simulink model "auto_pilot_udp"  (R2022b)
settings: Solver=FixedStepAuto  StartTime=0.0  StopTime=Inf  FixedStep=0.001  RelTol=1e-3  EnableMultiTasking=on
InitFcn:
  | clear mex
model workspace (MAT data in the model file):
  worldsim_instance.endpoint_ip = '127.0.0.1'
  worldsim_instance.endpoint_port = 8080
values from neighbouring files (symbols this model uses):
  ACC_Adaptive_D = 0    [AutoPilot_parameters.m]    (also in ap_ini_param.mat; ap_initialModel.sldd = 0.0)
  ACC_Adaptive_I = 0    [AutoPilot_parameters.m]    (also in ap_ini_param.mat; ap_initialModel.sldd = 0.0)
  ACC_Adaptive_P = [5 7.5]    [AutoPilot_parameters.m]    (also in ap_ini_param.mat; ap_initialModel.sldd = 5.0 7.5)
  ACC_Classic_I = 5    [AutoPilot_parameters.m]    (also in ap_ini_param.mat; ap_initialModel.sldd = 5.0)
  ACC_Classic_P = 15    [AutoPilot_parameters.m]    (also in ap_ini_param.mat; ap_initialModel.sldd = 15.0)
  ACC_MaxBrake = 50    [AutoPilot_parameters.m]    (also in ap_ini_param.mat; ap_initialModel.sldd = 50.0)
  ACC_MaxThrottle = 130    [AutoPilot_parameters.m]    (also in ap_ini_param.mat = 80; ap_initialModel.sldd = 130.0)
  ACC_Module_Activity_Flag = 1    [AutoPilot_parameters.m]    (also in ap_ini_param.mat; ap_initialModel.sldd = 1.0)
  ACC_Ready_Speed = 30    [AutoPilot_parameters.m]    (also in ap_ini_param.mat; ap_initialModel.sldd = 30.0)
  ACC_SensorMaxDistance = 250    [AutoPilot_parameters.m]    (also in ap_ini_param.mat = 120; ap_initialModel.sldd = 250.0)
  ACC_Speed_Distance_control = 3    [AutoPilot_parameters.m]    (also in ap_ini_param.mat; ap_initialModel.sldd = 3.0)
  ACC_Speed_Distance_Gain = [0.1 0.15 0.2 0.25]    [AutoPilot_parameters.m]    (also in ap_ini_param.mat; ap_initialModel.sldd = 0.1 0.15 0.2 0.25)
  ADAS_Control_Mode = 1    [AutoPilot_parameters.m]    (also in ap_ini_param.mat; ap_initialModel.sldd = 1.0)
  AEB_Alarm_Freq = 5    [AutoPilot_parameters.m]    (also in ap_ini_param.mat; ap_initialModel.sldd = 5.0)
  AEB_Distance_To_Collision_Brake = 5    [AutoPilot_parameters.m]    (also in ap_ini_param.mat; ap_initialModel.sldd = 5.0)
  AEB_Freq_Hz = Sensor_Freq_worldsim/2    (= 25)    [AutoPilot_parameters.m]    (also in ap_ini_param.mat; ap_initialModel.sldd = 25.0)
  AEB_Gain = [1 1]    [AutoPilot_parameters.m]    (also in ap_ini_param.mat; ap_initialModel.sldd = 1.0 1.0)
  AEB_Gain_set = 60    [AutoPilot_parameters.m]    (also in ap_ini_param.mat; ap_initialModel.sldd = 60.0)
  AEB_Gain_set_mult = 0.03    [AutoPilot_parameters.m]    (also in ap_ini_param.mat; ap_initialModel.sldd)
  AEB_Max_Decel = [8 15]    [AutoPilot_parameters.m]    (also in ap_ini_param.mat; ap_initialModel.sldd = 8.0 15.0)
  AEB_Max_Speed = 150    [AutoPilot_parameters.m]    (also in ap_ini_param.mat = 100; ap_initialModel.sldd = 150.0)
  AEB_Min_Distance_at_Stop = 1    [AutoPilot_parameters.m]    (also in ap_ini_param.mat; ap_initialModel.sldd = 1.0)
  AEB_Module_Activity_Flag = 1    [AutoPilot_parameters.m]    (also in ap_ini_param.mat; ap_initialModel.sldd = 1.0)
  AEB_Pedestrian_type = 68    [AutoPilot_parameters.m]    (also in ap_ini_param.mat; ap_initialModel.sldd = 68.0)
  AEB_Steer_Max = 180    [AutoPilot_parameters.m]    (also in ap_ini_param.mat; ap_initialModel.sldd = 180.0)
  AP_Activity_Flag = 1    [AutoPilot_parameters.m]    (also in ap_ini_param.mat; ap_initialModel.sldd = 1.0)
  AP_D = [0.3 0.3]    [AutoPilot_parameters.m]    (also in ap_ini_param.mat; ap_initialModel.sldd = 0.3 0.3)
  AP_Dyn_Rate_Limiter_Gain = 0.1    [AutoPilot_parameters.m]    (also in ap_ini_param.mat; ap_initialModel.sldd)
  AP_Dyn_Rate_Limiter_Power = 10    [AutoPilot_parameters.m]    (also in ap_ini_param.mat; ap_initialModel.sldd = 10.0)
  AP_Error_Max = 3    [AutoPilot_parameters.m]    (also in ap_ini_param.mat; ap_initialModel.sldd = 3.0)
  AP_Freq_Hz = Sensor_Freq_worldsim    (= 50)    [AutoPilot_parameters.m]    (also in ap_ini_param.mat; ap_initialModel.sldd = 50.0)
  AP_I = [0.05 0.05]    [AutoPilot_parameters.m]    (also in ap_ini_param.mat; ap_initialModel.sldd = 0.05 0.05)
  AP_Max_Error_dydt_Disable = 0.5    [AutoPilot_parameters.m]    (also in ap_ini_param.mat; ap_initialModel.sldd)
  AP_On_Request_Time = 0.01    [AutoPilot_parameters.m]    (also in ap_ini_param.mat; ap_initialModel.sldd)
  AP_P = [0.2 0.2]    [AutoPilot_parameters.m]    (also in ap_ini_param.mat; ap_initialModel.sldd = 0.2 0.2)
  AP_Steer_Error_Max = 0.7    [AutoPilot_parameters.m]    (also in ap_ini_param.mat; ap_initialModel.sldd)
  AP_Steer_Rate_Max_radps = 1    [AutoPilot_parameters.m]    (also in ap_ini_param.mat; ap_initialModel.sldd = 1.0)
  AP_Transition_Rate = 0.5    [AutoPilot_parameters.m]    (also in ap_ini_param.mat; ap_initialModel.sldd)
  butter_a = [1 -1.9911142922 0.991153595869]    [ap_ini_param.mat]    (also in ap_initialModel.sldd = 1.0 -1.9911142922016536 0.99115359586893548)
  butter_a_lka_out = 1.0 -1.5610180758007179 0.641351538057563    [ap_initialModel.sldd]
  butter_b = [9.82591682048e-06 1.9651833641e-05 9.82591682048e-06]    [ap_ini_param.mat]    (also in ap_initialModel.sldd = 9.825916820482009E-6 1.9651833640964018E-5 9.825916820482009)
  butter_b_lka_out = 0.020083365564211246 0.040166731128422492 0.020083365564211246    [ap_initialModel.sldd]
  Lane_Width = 3.7    [AutoPilot_parameters.m]    (also in ap_ini_param.mat; ap_initialModel.sldd)
  LDW_Activity_Flag = 1    [ap_ini_param.mat]    (also in ap_initialModel.sldd = 1.0)
  LDW_Freq_Hz = 50    [ap_ini_param.mat]    (also in ap_initialModel.sldd = 50.0)
  LDW_LaneGap_dydt_Warning = 50    [ap_ini_param.mat]    (also in ap_initialModel.sldd = 50.0)
  LDW_LaneGap_Warning = [0.5 0.25]    [ap_ini_param.mat]    (also in ap_initialModel.sldd = 0.5 0.25)
  LDW_Min_Speed = 60    [ap_ini_param.mat]    (also in ap_initialModel.sldd = 60.0)
  LDW_Steer_Vibration_Amplitude = 5    [ap_ini_param.mat]    (also in ap_initialModel.sldd = 5.0)
  LDW_Steer_Vibration_Freq = 25    [ap_ini_param.mat]    (also in ap_initialModel.sldd = 25.0)
  LKA_Activity_Flag = 1    [ap_ini_param.mat]    (also in ap_initialModel.sldd = 1.0)
  LKA_D = [0.2 0.3]    [ap_ini_param.mat]    (also in ap_initialModel.sldd = 0.2 0.3)
  LKA_Dyn_Rate_Limiter_Gain = 0.1    [ap_ini_param.mat]    (also in ap_initialModel.sldd)
  LKA_Dyn_Rate_Limiter_Power = 10    [ap_ini_param.mat]    (also in ap_initialModel.sldd = 10.0)
  LKA_Error_dydt_Off = 1    [ap_ini_param.mat]    (also in ap_initialModel.sldd = 1.0)
  LKA_Error_Max = 3    [ap_ini_param.mat]    (also in ap_initialModel.sldd = 3.0)
  LKA_Error_Off = 0.5    [ap_ini_param.mat]    (also in ap_initialModel.sldd)
  LKA_Freq_Hz = 50    [ap_ini_param.mat]    (also in ap_initialModel.sldd = 50.0)
  LKA_I = [0.025 0.05]    [ap_ini_param.mat]    (also in ap_initialModel.sldd = 0.025 0.05)
  LKA_Lane_Gap_Activate = [0.25 0.125]    [ap_ini_param.mat]    (also in ap_initialModel.sldd = 0.25 0.125)
  LKA_Lane_Gap_dydt_Activate = 50    [ap_ini_param.mat]    (also in ap_initialModel.sldd = 50.0)
  LKA_Min_Speed = 60    [ap_ini_param.mat]    (also in ap_initialModel.sldd = 60.0)
  LKA_On_Display_Freq = 5    [ap_ini_param.mat]    (also in ap_initialModel.sldd = 5.0)
  LKA_P = [0.1 0.2]    [ap_ini_param.mat]    (also in ap_initialModel.sldd = 0.1 0.2)
  LKA_Steer_Rate_Max_radps = 1    [ap_ini_param.mat]    (also in ap_initialModel.sldd = 1.0)
  No_Target_Display_Value = 0    [AutoPilot_parameters.m]    (also in ap_ini_param.mat; ap_initialModel.sldd = 0.0)
  radar_source = 2    [AutoPilot_parameters.m]    (also in ap_ini_param.mat; ap_initialModel.sldd = 2.0)
  Sensor_Freq_worldsim = 50    [AutoPilot_parameters.m]    (also in ap_ini_param.mat; ap_initialModel.sldd = 50.0; launcher.m)
  stop_number_collisions = 10.0    [ap_initialModel.sldd]    (also in launcher.m = 10)
  stop_speed = 0.001    [ap_initialModel.sldd]    (also in launcher.m)
  stop_time = 12.0    [ap_initialModel.sldd]    (also in launcher.m = 12)
  vehicle_width = 2.2    [AutoPilot_parameters.m]    (also in ap_ini_param.mat = 1.86; ap_initialModel.sldd)
undefined symbols (not defined in the file or in its folder): blockPlatform, HOST, light_brake_center, light_brake_left, light_brake_right
libraries: simulink x103, simwbSfunlib x35, slpidlib x5, viworldsim_lib x5
(part 1 of 5)
settings Model: DataDictionary=ap_initialModel.sldd  Creator=mcava  LastModifiedBy=pumpaipa
settings SolverCC: AlgebraicLoopSolver=TrustRegion  AutoInsertRateTranBlk=on
settings DataIOCC: LimitDataPoints=on  SaveFormat=Array  ReturnWorkspaceOutputs=off  SignalLoggingName=sigsOut
settings OptimizationCC: ExpressionDepthLimit=2147483647  InitFltsAndDblsToZero=on
settings DebuggingCC: SignalInfNanChecking=warning  UnderspecifiedInitializationDetection=Classic  MergeDetectMultiDrivingBlocksExec=none  SignalResolutionControl=TryResolveAllWithWarning  MultiTaskDSMMsg=warning  MultiTaskCondExecSysMsg=none  FcnCallInpInsideContextMsg=warning  UnconnectedInputMsg=warning  UnconnectedOutputMsg=warning  UnconnectedLineMsg=warning  StateNameClashWarn=warning  SFUnexpectedBacktrackingDiag=warning  SFNoUnconditionalDefaultTransitionDiag=warning  SFExecutionAtInitializationDiag=none  SFMachineParentedDataDiag=warning  ArithmeticOperatorsInVariantConditions=warning
settings HardwareCC: ProdBitPerLong=64  ProdHWDeviceType=Intel->x86-64 (Linux 64)  TargetHWDeviceType=32-bit Generic
settings ModelReferenceCC: EnableRefExpFcnMdlSchedulingChecks=on  PropagateSignalLabelsOutOfModel=off
settings SFSimCC: SimUseLocalCustomCode=off  CustomCodeUndefinedFunction=UseInterfaceOnly
settings RTWCC: Description=VI-CarRealTime Solver Plugin V1.0  SystemTargetFile=vicrt_plugin.tlc  GenCodeOnly=on  PackageGeneratedCodeAndArtifacts=on  TemplateMakefile=vicrt_plugin_ccur.tmf  PostCodeGenCommand=if strcmp(get_param(bdroot,'TemplateMakefile'),'vicrt_plugin_ccur.tmf'),copyfile([matlabroot,filesep,'rtw',filesep,'c',filesep,'tools',filesep,'unixtools.mk'],'unixtools.mk'),if ~verLessThan('matlab','9.6'),set_param(bdroot,'MatFileLogging','off'),end,end  RTWUseLocalCustomCode=off
settings CodeAppCC: MaxIdLength=80  StateflowObjectComments=on
settings STFCustomTargetCC: ModelReferenceCompliant=off  CombineOutputUpdateFcns=on  SystemTargetFile=vicrt_plugin.tlc
settings GRTTargetCC: TargetLangStandard=C89/C90 (ANSI)  ModelReferenceCompliant=off  ParMdlRefBuildCompliant=off  CompOptLevelCompliant=off  ConcurrentExecutionCompliant=off  MatFileLogging=off  CPPClassGenCompliant=off  UseToolchainInfoCompliant=off  RTWCAPIParams=on
settings ConfigComp: CovMetricSettings=dw  CovSaveCumulativeToWorkspaceVar=on  CovSaveSingleToWorkspaceVar=on  CovExternalEMLEnable=off

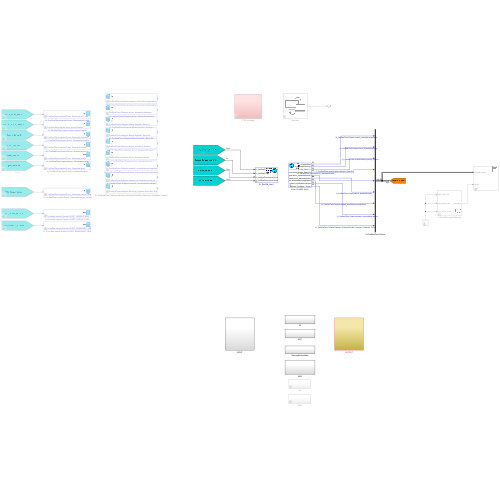
[thumbnail: Simulink's stored preview of the top-level diagram]
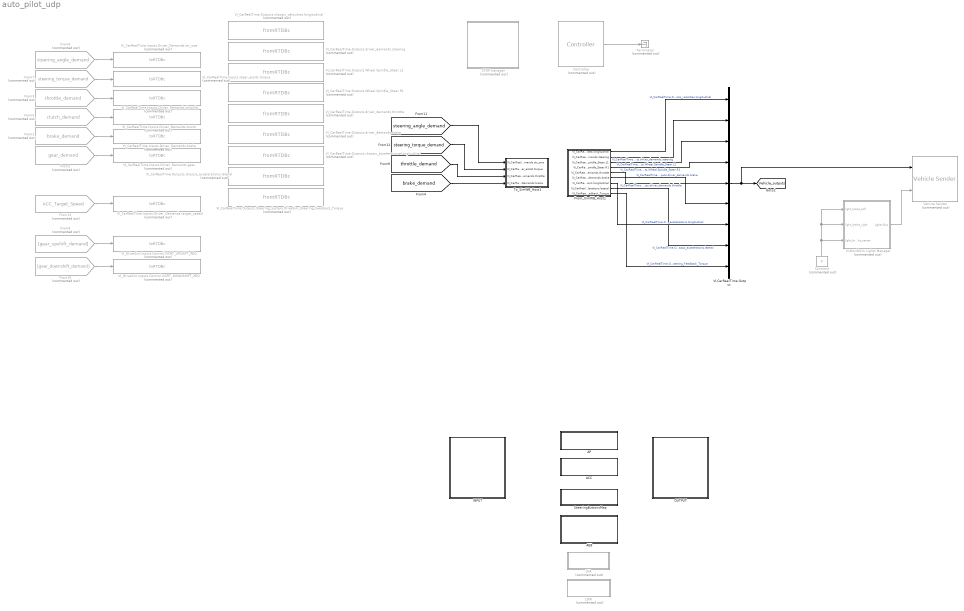
== system auto_pilot_udp ==
  ACC : Subsystem
  AEB : Subsystem
  AP : Subsystem
  Constant : Constant  Commented=on  Value=0
  Controller : viworldsim_lib/Controller  Commented=on  worldsim_endpoint_ip=worldsim_instance.endpoint_ip  worldsim_endpoint_port=worldsim_instance.endpoint_port  worldsim_verbose=off
  From1 : From  Commented=on  GotoTag=brake_demand  TagVisibility=global
  From10 : From  Commented=on  GotoTag=gear_downshift_demand  TagVisibility=global
  From13 : From  Commented=on  GotoTag=ACC_Target_Speed  TagVisibility=global
  From2 : From  Commented=on  GotoTag=gear_demand  TagVisibility=global
  From3 : From  Commented=on  GotoTag=throttle_demand  TagVisibility=global
  From5 : From  Commented=on  GotoTag=clutch_demand  TagVisibility=global
  From6 : From  Commented=on  GotoTag=steering_angle_demand  TagVisibility=global
  From7 : From  Commented=on  GotoTag=steering_torque_demand  TagVisibility=global
  From8 : From  Commented=on  GotoTag=gear_upshift_demand  TagVisibility=global
  From_SimWB_Host1 : Subsystem  mask(From_SimWB_Host){numPorts=9, inheritPortNames=off, portNames={'VI_CarRealTime.Outputs.chassis_velocities.longitudinal','VI_CarRealTime.Outputs.driver_demands.steering','VI_CarRealTime.Outputs.Wheel.Spindle_Steer.L1','VI_CarRealTime.Outputs.Wheel.Spindle_Steer.R1','VI_CarRealTime.Outputs.driver_demands.throttle','VI_CarRealTime.Outputs.driver_demands.brake','VI_CarRealTime.Outputs.chassis_accelerations.longitudinal','VI_CarRealTime.Outputs.chassis_accelerations.lateral','VI_CarRealTime.Outputs.Steering_System.DriveSim_Steering_Feedback_Torque'}, origNumPorts=1, blockCode=6578738372in, localIP='192.168.100.150', localPort=25000, remoteURL='192.168.100.20', recvBufferSize=72, dims=72, blockingTime=0, sampletime=0.01, signalDatatype=uint8, isVarSize=off, blockPlatform=blockPlatform, isComplex=on, msk_dimensions={1,1,1,1,1,1,1,1,1}, msk_datatypes={'double','double','double','double','double','double','double','double','double'}, byteAlign=1}
      mask prompts: numPorts "Number of Ports:"; inheritPortNames "Inherit Port Names:"; portNames "Port Names: {'a','b','c'}"; origNumPorts "Orig Num"; blockCode "Block Code"; localIP "Local IP address (SimWB sends data to this IP)"; localPort "Local IP port:"; remoteURL "Remote IP address ('0.0.0.0' to accept all):"; recvBufferSize "Receive buffer size (bytes):"; dims "Maximum length for Message:"; blockingTime "Blocking time (seconds):"; sampletime "Sample time (seconds):"; signalDatatype "Data type for Message:"; isVarSize "Output variable-size signal"; blockPlatform "Block Platform:"; isComplex "Message is Complex"; msk_dimensions "Output port dimensions:"; msk_datatypes "Output port data type:"; byteAlign "Byte alignment:"
      mask help: This block receives UDP packets from the specified SimWB host. This block is supported in MATLAB R2011a and later only.
      mask init:
      | set_param(gcbh,'blockCode','6578738372in');
      mask Help: web([simwbroot 'html' filesep 'simwb_blocks_udp.html'])
      mask Callback numPorts: UDPBlockSetup(gcbh,'INPUT');
      mask Callback inheritPortNames:
      | maskVisibilities =  get_param(gcbh,'MaskVisibilities');
      | if  strcmp(get_param(gcbh,'inheritPortNames'),'on')
      |     maskVisibilities{3} = 'off';
      | else
      |     maskVisibilities{3} = 'on';
      | end
      | set_param(gcbh,'MaskVisibilities',maskVisibilities);
      mask Callback portNames: UDPBlockSetup(gcbh,'UPDATEOUTPORTNAMES');
      mask Callback msk_dimensions: UDPBlockSetup(gcbh,'BYTEUNPACKCHANGED');
      mask Callback msk_datatypes: UDPBlockSetup(gcbh,'BYTEUNPACKCHANGED');
      mask DialogControl ParameterTabVar0 Prompt: General
      mask DialogControl ParameterTabVar01 Prompt: UDP
      mask DialogControl ParameterTabVar012 Prompt: Byte Unpack
      mask Display: image(imread('udpreceive.png'),'top-left')
  INPUT : Subsystem
  LDW : Subsystem  Commented=on
  LKA : Subsystem  Commented=on
  OUTPUT : Subsystem
  STOP manager : Subsystem  Commented=on
  SteeringButtonsMap : Subsystem
  Terminator : Terminator  Commented=on
  To_SimWB_Host1 : Subsystem  mask(To_SimWB_Host){numPorts=4, inheritPortNames=off, portNames={'VI_CarRealTime.Inputs.Driver_Demands.str_swa','VI_CarRealTime.Inputs.steer_assist.torque','VI_CarRealTime.Inputs.Driver_Demands.throttle','VI_CarRealTime.Inputs.Driver_Demands.brake'}, remoteURL='255.255.255.255', remotePort=25001, blockPlatform=HOST, msk_datatypes={'double','double','double','double'}, byteAlign=1, origNumPorts=1, blockCode=6578738372out, sendBufferSize=8192}
      mask prompts: numPorts "Number of Ports:"; inheritPortNames "Inherit Port Names:"; portNames "Port Names: {'a','b','c'}"; remoteURL "Remote IP address ('255.255.255.255' for broadcast):"; remotePort "Remote IP port:"; blockPlatform "Block Platform"; msk_datatypes "Input port data types (cell array):"; byteAlign "Byte alignment:"; origNumPorts "Orig Num"; blockCode "Block Code"; sendBufferSize "Send Buffer Size"
      mask help: This block sends UDP packets to the specified SimWB host. This block is supported in MATLAB R2011a and later only.
      mask Help: web([simwbroot 'html' filesep 'simwb_blocks_udp.html']);
      mask Callback numPorts: UDPBlockSetup(gcbh,'OUTPUT');
      mask Callback inheritPortNames:
      | maskVisibilities =  get_param(gcbh,'MaskVisibilities');
      | if  strcmp(get_param(gcbh,'inheritPortNames'),'on')
      |     maskVisibilities{3} = 'off';
      | else
      |     maskVisibilities{3} = 'on';
      | end
      | set_param(gcbh,'MaskVisibilities',maskVisibilities);
      mask Callback portNames: UDPBlockSetup(gcbh,'UPDATEINPORTNAMES');
      mask Callback msk_datatypes: UDPBlockSetup(gcbh,'BYTEPACKCHANGED');
      mask DialogControl ParameterTabVar0 Prompt: General
      mask DialogControl ParameterTabVar01 Prompt: UDP
      mask DialogControl ParameterTabVar012 Prompt: Byte Pack
      mask Display: image(imread('udpsend.png'),'top-right')
  VI-CarRealTime.Output : BusCreator  Inputs=9
  VI-WorldSim Lights Manager : Subsystem  Commented=on  mask{DummyMaskPar=0}
      mask init:
      | set_param(gcb, 'LinkStatus','none')
      settings: OpenFcn=|
      | wsoffline_lightsmanager;
      | set_param(gcb, 'LinkStatus','none');
      mask Display:
      | color('black');
      | image('lights.png', [85 0 50 50]);
  VI_CarRealTime.Inputs.Driver_Demands.brake : simwbSfunlib/toRTDBc  Commented=on  stringBlock=off  varName=VI_CarRealTime.Inputs.Driver_Demands.brake  sigDim=[1 1]  sigType=double  sampleTime=[-1 0]  maxBuffSize=1024  busName=nobus  defaultValue=0  defaultString=simwbout  hasMapping=0  ptrName=VI_CarRealTime_Inputs_Driver_Demands_brake  enumOrAlias=nothing
      settings: SourceProductName=SimWB MLToolkit
  VI_CarRealTime.Inputs.Driver_Demands.clutch : simwbSfunlib/toRTDBc  Commented=on  stringBlock=off  varName=VI_CarRealTime.Inputs.Driver_Demands.clutch  sigDim=[1 1]  sigType=double  sampleTime=[-1 0]  maxBuffSize=1024  busName=nobus  defaultValue=0  defaultString=simwbout  hasMapping=0  ptrName=VI_CarRealTime_Inputs_Driver_Demands_clutch  enumOrAlias=nothing
      settings: SourceProductName=SimWB MLToolkit
  VI_CarRealTime.Inputs.Driver_Demands.gear : simwbSfunlib/toRTDBc  Commented=on  stringBlock=off  varName=VI_CarRealTime.Inputs.Driver_Demands.gear  sigDim=[1 1]  sigType=double  sampleTime=[-1 0]  maxBuffSize=1024  busName=nobus  defaultValue=0  defaultString=simwbout  hasMapping=0  ptrName=VI_CarRealTime_Inputs_Driver_Demands_gear  enumOrAlias=nothing
      settings: SourceProductName=SimWB MLToolkit
  VI_CarRealTime.Inputs.Driver_Demands.str_swa : simwbSfunlib/toRTDBc  Commented=on  stringBlock=off  varName=VI_CarRealTime.Inputs.Driver_Demands.str_swa  sigDim=[1 1]  sigType=double  sampleTime=[-1 0]  maxBuffSize=1024  busName=nobus  defaultValue=0  defaultString=simwbout  hasMapping=0  ptrName=VI_CarRealTime_Inputs_Driver_Demands_str_swa  enumOrAlias=nothing
      settings: SourceProductName=SimWB MLToolkit
  VI_CarRealTime.Inputs.Driver_Demands.target_speed : simwbSfunlib/toRTDBc  Commented=on  stringBlock=off  varName=VI_CarRealTime.Inputs.Driver_Demands.target_speed  sigDim=[1 1]  sigType=double  sampleTime=[-1 0]  maxBuffSize=1024  busName=nobus  defaultValue=0  defaultString=simwbout  hasMapping=0  ptrName=VI_CarRealTime_Inputs_Driver_Demands_target_speed  enumOrAlias=nothing
      settings: SourceProductName=SimWB MLToolkit
  VI_CarRealTime.Inputs.Driver_Demands.throttle : simwbSfunlib/toRTDBc  Commented=on  stringBlock=off  varName=VI_CarRealTime.Inputs.Driver_Demands.throttle  sigDim=[1 1]  sigType=double  sampleTime=[-1 0]  maxBuffSize=1024  busName=nobus  defaultValue=0  defaultString=simwbout  hasMapping=0  ptrName=VI_CarRealTime_Inputs_Driver_Demands_throttle  enumOrAlias=nothing
      settings: SourceProductName=SimWB MLToolkit
  VI_CarRealTime.Inputs.steer_assist.torque : simwbSfunlib/toRTDBc  Commented=on  stringBlock=off  varName=VI_CarRealTime.Inputs.steer_assist.torque  sigDim=[1 1]  sigType=double  sampleTime=[-1 0]  maxBuffSize=1024  busName=nobus  defaultValue=0  defaultString=simwbout  hasMapping=0  ptrName=VI_CarRealTime_Inputs_steer_assist_torque  enumOrAlias=nothing
      settings: SourceProductName=SimWB MLToolkit
  VI_CarRealTime.Outputs.Steering_System.DriveSim_Steering_Feedback_Torque : simwbSfunlib/fromRTDBc  Commented=on  stringBlock=off  varName=VI_CarRealTime.Outputs.Steering_System.DriveSim_Steering_Feedback_Torque  sigDim=[1 1]  sigType=double  sampleTime=[-1 0]  maxBuffSize=1024  busName=nobus  defaultValue=0  defaultString=simwbin  hasMapping=0  ptrName=VI_CarRealTime_Outputs_Steering_System_DriveSim_Steering_Feedback_Torque  enumOrAlias=nothing
      settings: SourceProductName=SimWB MLToolkit
  VI_CarRealTime.Outputs.Wheel.Spindle_Steer.L1 : simwbSfunlib/fromRTDBc  Commented=on  stringBlock=off  varName=VI_CarRealTime.Outputs.Wheel.Spindle_Steer.L1  sigDim=[1 1]  sigType=double  sampleTime=[-1 0]  maxBuffSize=1024  busName=nobus  defaultValue=0  defaultString=simwbin  hasMapping=0  ptrName=VI_CarRealTime_Outputs_Wheel_Spindle_Steer_L1  enumOrAlias=nothing
      settings: SourceProductName=SimWB MLToolkit
  VI_CarRealTime.Outputs.Wheel.Spindle_Steer.R1 : simwbSfunlib/fromRTDBc  Commented=on  stringBlock=off  varName=VI_CarRealTime.Outputs.Wheel.Spindle_Steer.R1  sigDim=[1 1]  sigType=double  sampleTime=[-1 0]  maxBuffSize=1024  busName=nobus  defaultValue=0  defaultString=simwbin  hasMapping=0  ptrName=VI_CarRealTime_Outputs_Wheel_Spindle_Steer_R1  enumOrAlias=nothing
      settings: SourceProductName=SimWB MLToolkit
  VI_CarRealTime.Outputs.chassis_accelerations.lateral : simwbSfunlib/fromRTDBc  Commented=on  stringBlock=off  varName=VI_CarRealTime.Outputs.chassis_accelerations.lateral  sigDim=[1 1]  sigType=double  sampleTime=[-1 0]  maxBuffSize=1024  busName=nobus  defaultValue=0  defaultString=simwbin  hasMapping=0  ptrName=VI_CarRealTime_Outputs_chassis_accelerations_lateral  enumOrAlias=nothing
      settings: SourceProductName=SimWB MLToolkit
  VI_CarRealTime.Outputs.chassis_accelerations.longitudinal : simwbSfunlib/fromRTDBc  Commented=on  stringBlock=off  varName=VI_CarRealTime.Outputs.chassis_accelerations.longitudinal  sigDim=[1 1]  sigType=double  sampleTime=[-1 0]  maxBuffSize=1024  busName=nobus  defaultValue=0  defaultString=simwbin  hasMapping=0  ptrName=VI_CarRealTime_Outputs_chassis_accelerations_longitudinal  enumOrAlias=nothing
      settings: SourceProductName=SimWB MLToolkit
  VI_CarRealTime.Outputs.chassis_velocities.longitudinal : simwbSfunlib/fromRTDBc  Commented=on  stringBlock=off  varName=VI_CarRealTime.Outputs.chassis_velocities.longitudinal  sigDim=[1 1]  sigType=double  sampleTime=[-1 0]  maxBuffSize=1024  busName=nobus  defaultValue=0  defaultString=simwbin  hasMapping=0  ptrName=VI_CarRealTime_Outputs_chassis_velocities_longitudinal  enumOrAlias=nothing
      settings: SourceProductName=SimWB MLToolkit
  VI_CarRealTime.Outputs.driver_demands.brake : simwbSfunlib/fromRTDBc  Commented=on  stringBlock=off  varName=VI_CarRealTime.Outputs.driver_demands.brake  sigDim=[1 1]  sigType=double  sampleTime=[-1 0]  maxBuffSize=1024  busName=nobus  defaultValue=0  defaultString=simwbin  hasMapping=0  ptrName=VI_CarRealTime_Outputs_driver_demands_brake  enumOrAlias=nothing
      settings: SourceProductName=SimWB MLToolkit
  VI_CarRealTime.Outputs.driver_demands.steering : simwbSfunlib/fromRTDBc  Commented=on  stringBlock=off  varName=VI_CarRealTime.Outputs.driver_demands.steering  sigDim=[1 1]  sigType=double  sampleTime=[-1 0]  maxBuffSize=1024  busName=nobus  defaultValue=0  defaultString=simwbin  hasMapping=0  ptrName=VI_CarRealTime_Outputs_driver_demands_steering  enumOrAlias=nothing
      settings: SourceProductName=SimWB MLToolkit
  VI_CarRealTime.Outputs.driver_demands.throttle : simwbSfunlib/fromRTDBc  Commented=on  stringBlock=off  varName=VI_CarRealTime.Outputs.driver_demands.throttle  sigDim=[1 1]  sigType=double  sampleTime=[-1 0]  maxBuffSize=1024  busName=nobus  defaultValue=0  defaultString=simwbin  hasMapping=0  ptrName=VI_CarRealTime_Outputs_driver_demands_throttle  enumOrAlias=nothing
      settings: SourceProductName=SimWB MLToolkit
  VI_DriveSim.Inputs.Control.VICRT_DOWNSHIFT_REQ : simwbSfunlib/toRTDBc  Commented=on  stringBlock=off  varName=VI_DriveSim.Inputs.Control.VICRT_DOWNSHIFT_REQ  sigDim=[1 1]  sigType=double  sampleTime=[-1 0]  maxBuffSize=1024  busName=nobus  defaultValue=0  defaultString=simwbout  hasMapping=0  ptrName=VI_DriveSim_Inputs_Control_VICRT_DOWNSHIFT_REQ  enumOrAlias=nothing
      settings: SourceProductName=SimWB MLToolkit
  VI_DriveSim.Inputs.Control.VICRT_UPSHIFT_REQ : simwbSfunlib/toRTDBc  Commented=on  stringBlock=off  varName=VI_DriveSim.Inputs.Control.VICRT_UPSHIFT_REQ  sigDim=[1 1]  sigType=double  sampleTime=[-1 0]  maxBuffSize=1024  busName=nobus  defaultValue=0  defaultString=simwbout  hasMapping=0  ptrName=VI_DriveSim_Inputs_Control_VICRT_UPSHIFT_REQ  enumOrAlias=nothing
      settings: SourceProductName=SimWB MLToolkit
  Vehicle Sender : viworldsim_lib/VI-WorldSim Vehicle Senders/Vehicle Sender  Commented=on  useOutputMapInMaskFlag=on  worldsim_car_name='ego'  worldsim_ai_controlled=off
      link override VI_WorldSim_VehicleSender: worldsim_car_name='ego'
  tag scope: Vehicle_outputs=global
  wires:
  From3/1 -> VI_CarRealTime.Inputs.Driver_Demands.throttle/1
  From5/1 -> VI_CarRealTime.Inputs.Driver_Demands.clutch/1
  From6/1 -> VI_CarRealTime.Inputs.Driver_Demands.str_swa/1
  From7/1 -> VI_CarRealTime.Inputs.steer_assist.torque/1
  From1/1 -> VI_CarRealTime.Inputs.Driver_Demands.brake/1
  From2/1 -> VI_CarRealTime.Inputs.Driver_Demands.gear/1
  Controller/1 -> Terminator/1
  Constant/1 -> VI-WorldSim Lights Manager/3(light_brake_center), VI-WorldSim Lights Manager/2(light_brake_right), VI-WorldSim Lights Manager/1(light_brake_left)
  VI-WorldSim Lights Manager/1(Lights Bus) -> Vehicle Sender/2
  From_SimWB_Host1/1(VI_CarRealTime.Outputs.chassis_velocities.longitudinal) -> VI-CarRealTime.Output/1  "VI_CarRealTime.Outputs.chassis_velocities.longitudinal"
  From_SimWB_Host1/2(VI_CarRealTime.Outputs.driver_demands.steering) -> VI-CarRealTime.Output/2  "VI_CarRealTime.Outputs.driver_demands.steering"
  From_SimWB_Host1/3(VI_CarRealTime.Outputs.Wheel.Spindle_Steer.L1) -> VI-CarRealTime.Output/3  "VI_CarRealTime.Outputs.Wheel.Spindle_Steer.L1"
  From_SimWB_Host1/4(VI_CarRealTime.Outputs.Wheel.Spindle_Steer.R1) -> VI-CarRealTime.Output/4  "VI_CarRealTime.Outputs.Wheel.Spindle_Steer.R1"
  From_SimWB_Host1/6(VI_CarRealTime.Outputs.driver_demands.brake) -> VI-CarRealTime.Output/6  "VI_CarRealTime.Outputs.driver_demands.brake"
  From_SimWB_Host1/5(VI_CarRealTime.Outputs.driver_demands.throttle) -> VI-CarRealTime.Output/5  "VI_CarRealTime.Outputs.driver_demands.throttle"
  From_SimWB_Host1/7(VI_CarRealTime.Outputs.chassis_accelerations.longitudinal) -> VI-CarRealTime.Output/7  "VI_CarRealTime.Outputs.chassis_accelerations.longitudinal"
  From_SimWB_Host1/8(VI_CarRealTime.Outputs.chassis_accelerations.lateral) -> VI-CarRealTime.Output/8  "VI_CarRealTime.Outputs.chassis_accelerations.lateral"
  From_SimWB_Host1/9(VI_CarRealTime.Outputs.Steering_System.DriveSim_Steering_Feedback_Torque) -> VI-CarRealTime.Output/9  "VI_CarRealTime.Outputs.Steering_System.DriveSim_Steering_Feedback_Torque"
  VI-CarRealTime.Output/1 -> Vehicle Sender/1, [Vehicle_outputs]
  [steering_angle_demand] -> To_SimWB_Host1/1(VI_CarRealTime.Inputs.Driver_Demands.str_swa)
  [steering_torque_demand] -> To_SimWB_Host1/2(VI_CarRealTime.Inputs.steer_assist.torque)
  [throttle_demand] -> To_SimWB_Host1/3(VI_CarRealTime.Inputs.Driver_Demands.throttle)
  [brake_demand] -> To_SimWB_Host1/4(VI_CarRealTime.Inputs.Driver_Demands.brake)
  From8/1 -> VI_DriveSim.Inputs.Control.VICRT_UPSHIFT_REQ/1
  From13/1 -> VI_CarRealTime.Inputs.Driver_Demands.target_speed/1
  From10/1 -> VI_DriveSim.Inputs.Control.VICRT_DOWNSHIFT_REQ/1

== system auto_pilot_udp/ACC ==
  ACC_Inputs : Subsystem
  ACC_Logic : Subsystem
  ACC_Outputs : Subsystem

== system auto_pilot_udp/AEB ==
  AEB_Inputs : Subsystem
  AEB_Logic : Subsystem
  AEB_Outputs : Subsystem

== system auto_pilot_udp/AP ==
  AP_Inputs : Subsystem
  AP_Logic : Subsystem
  AP_Outputs : Subsystem

== system auto_pilot_udp/From_SimWB_Host1 ==
  Byte Unpack : S-Function  FunctionName=byte2any  Parameters=dimensionsout, datatypesout, byteAlign  SFunctionDeploymentMode=off  EnableBusSupport=off  mask(Byte Unpack){dimensions={1,1,1,1,1,1,1,1,1}, datatypes={'double','double','double','double','double','double','double','double','double'}, byteAlign=1}
      mask prompts: dimensions "Output port dimensions (cell array):"; datatypes "Output port data types (cell array):"; byteAlign "Byte alignment:"
      mask help: Unpack a binary byte vector to extract data. Insert after a UDP Recv block to break-up a UDP packet into its constituent data vectors.
      mask init:
      | [dimensionsout, datatypesout]= byteunpack_callback(dimensions, datatypes);
      mask Help: eval('linkfoundation.util.blockHelpLink(''ecoder'')');
      mask TypeOptions byteAlign: 1 | 2 | 4 | 8
      mask Display:
      | color('blue');
      | text(0.95, 0.90, '', ...
      |                 'horizontalalignment', 'right');
      | color('black');
      | text(0.50, 0.12, 'Byte Unpack', ...
      |                 'horizontalAlignment','center');
  Term : Terminator
  UDP Receive : S-Function  FunctionName=sdspFromNetwork  Parameters=localURL, localPort, remoteURL, remotePort, recvBufferSize, signalDatatype, dims, sampletime, isVarSize, blockingTime, isComplex  SFunctionDeploymentMode=off  EnableBusSupport=off  mask(UDP Receive){localURL='0.0.0.0', localPort=localPort, remoteURL=remoteURL, remotePort=-1, recvBufferSize=recvBufferSize, dims=dims, signalDatatype=uint8, isComplex=off, isVarSize=off, showBlockingTime=on, blockingTime=blockingTime, sampletime=sampletime, blockPlatform=blockPlatform}
      mask prompts: localURL "Local IP address:"; localPort "Local IP port:"; remoteURL "Remote IP address ('0.0.0.0' to accept all):"; remotePort "Remote IP port:"; recvBufferSize "Receive buffer size (bytes):"; dims "Maximum length for Message:"; signalDatatype "Data type for Message:"; isComplex "Message is complex"; isVarSize "Output variable-size signal"; showBlockingTime "Show blocking time"; blockingTime "Blocking time (seconds):"; sampletime "Sample time (seconds):"; blockPlatform "Block Platform"
      mask help:
      | Receive UDP packets on a given IP port.
      | This block receives a UDP packet from the network and emits that data as a one-dimensional vector of the specified data type.
      mask init:
      | icon = sprintf('%s\n', 'fprintf(''UDP Receive'');');
      | % If there are multiple ports, label them
      | if strcmp(get_param(gcb,'isVarSize'), 'off')
      |     icon = sprintf('%s%s\n', icon, 'port_label(''output'', 1, ''Message'');');
      |     icon = sprintf('%s%s\n', icon, 'port_label(''output'', 2, ''Length'');');
      | end
      | icon = [icon sprintf('%s\n','color(''blue'');')];
      | icon = [icon sprintf('%s\n','text(0.97, 0.87, get_param(gcb, ''blockPlatform''), ''horizontalalignment'', ''right'');')];
      | set_param(gcb, 'maskDisplay', icon);
      | 
      | % Hide the lengthDatatype and BlockingTime if required
      | vis = get_param(gcbh, 'MaskVisibilities');
      | vis{10} = get_param(gcbh, 'showBlockingTime');
      | set_param(gcbh, 'MaskVisibilities', vis);
      mask Help: eval('dspnetwork_help(''UDPReceive'')')
      mask TypeOptions signalDatatype: double | single | int8 | uint8 | int16 | uint16 | int32 | uint32 | boolean
      mask Display:
      | fprintf('UDP Receive');
      | port_label('output', 1, 'Message');
      | port_label('output', 2, 'Length');
      | color('blue');
      | text(0.97, 0.87, get_param(gcb, 'blockPlatform'), 'horizontalalignment', 'right');
  VI_CarRealTime.Outputs.chassis_velocities.longitudinal : Outport
  VI_CarRealTime.Outputs.driver_demands.steering : Outport  Port=2
  VI_CarRealTime.Outputs.Wheel.Spindle_Steer.L1 : Outport  Port=3
  VI_CarRealTime.Outputs.Wheel.Spindle_Steer.R1 : Outport  Port=4
  VI_CarRealTime.Outputs.driver_demands.throttle : Outport  Port=5
  VI_CarRealTime.Outputs.driver_demands.brake : Outport  Port=6
  VI_CarRealTime.Outputs.chassis_accelerations.longitudinal : Outport  Port=7
  VI_CarRealTime.Outputs.chassis_accelerations.lateral : Outport  Port=8
  VI_CarRealTime.Outputs.Steering_System.DriveSim_Steering_Feedback_Torque : Outport  Port=9
  wires:
  UDP Receive/1 -> Byte Unpack/1
  UDP Receive/2 -> Term/1
  Byte Unpack/1 -> VI_CarRealTime.Outputs.chassis_velocities.longitudinal/1
  Byte Unpack/2 -> VI_CarRealTime.Outputs.driver_demands.steering/1
  Byte Unpack/3 -> VI_CarRealTime.Outputs.Wheel.Spindle_Steer.L1/1
  Byte Unpack/4 -> VI_CarRealTime.Outputs.Wheel.Spindle_Steer.R1/1
  Byte Unpack/5 -> VI_CarRealTime.Outputs.driver_demands.throttle/1
  Byte Unpack/6 -> VI_CarRealTime.Outputs.driver_demands.brake/1
  Byte Unpack/7 -> VI_CarRealTime.Outputs.chassis_accelerations.longitudinal/1
  Byte Unpack/8 -> VI_CarRealTime.Outputs.chassis_accelerations.lateral/1
  Byte Unpack/9 -> VI_CarRealTime.Outputs.Steering_System.DriveSim_Steering_Feedback_Torque/1

== system auto_pilot_udp/INPUT ==
  Inputs for CRT : Subsystem

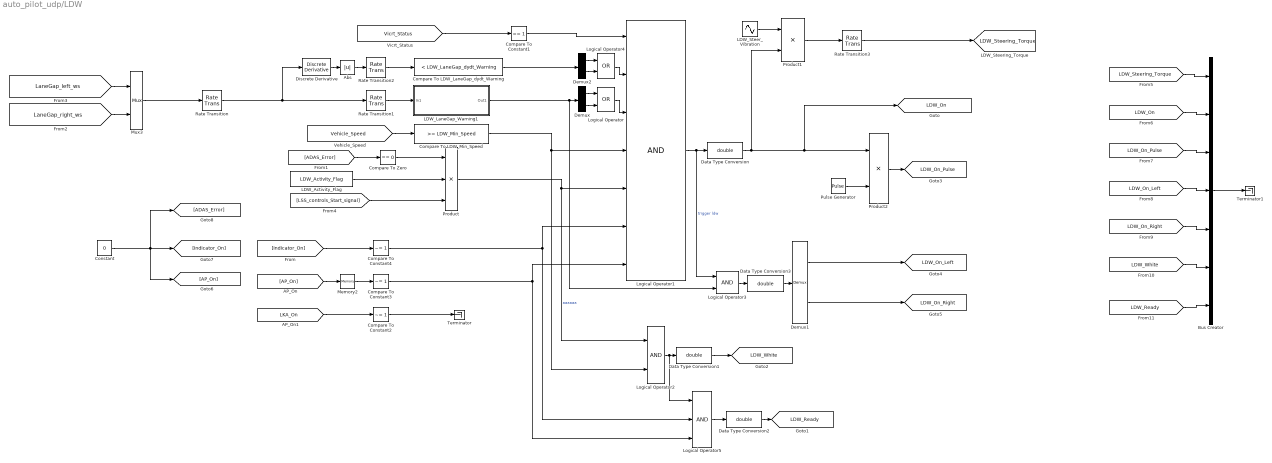
== system auto_pilot_udp/LDW ==
  Abs : Abs  SaturateOnIntegerOverflow=off
  Bus Creator : BusCreator  Inputs=7
  Compare To Constant1 : simulink/Logic and Bit Operations/Compare To Constant  relop===  const=1  OutDataTypeStr=boolean
  Compare To Constant2 : simulink/Logic and Bit Operations/Compare To Constant  relop=~=  const=1  OutDataTypeStr=boolean
  Compare To Constant3 : simulink/Logic and Bit Operations/Compare To Constant  relop=~=  const=1  OutDataTypeStr=boolean
  Compare To Constant4 : simulink/Logic and Bit Operations/Compare To Constant  relop=~=  const=1  OutDataTypeStr=boolean
  Compare To Zero : simulink/Logic and Bit Operations/Compare To Zero  relop===  OutDataTypeStr=boolean
  Compare To LDW_LaneGap_dydt_Warning : simulink/Logic and Bit Operations/Compare To Constant  relop=<  const=LDW_LaneGap_dydt_Warning  OutDataTypeStr=boolean
  Compare To LDW_Min_Speed : simulink/Logic and Bit Operations/Compare To Constant  relop=>=  const=LDW_Min_Speed  OutDataTypeStr=boolean
  Constant : Constant  Value=0
  Data Type Conversion{,1..3} (4 alike) : DataTypeConversion  OutDataTypeStr=double  SaturateOnIntegerOverflow=off  RndMeth=Floor
  Demux : Demux  Outputs=2
  Demux1 : Demux  Outputs=2
  Demux2 : Demux  Outputs=2
  Discrete Derivative : simulink/Discrete/Discrete Derivative  gainval=1.0  ICPrevScaledInput=0.0  OutMin=[]  OutMax=[]  OutDataType=fixdt(1, 16)  OutScaling=2^-10  DoSatur=off
  LDW_Activity_Flag : Constant  Value=LDW_Activity_Flag
  LDW_LaneGap_Warning1 : Subsystem
  LDW_Steer_Vibration : Sin  Amplitude=LDW_Steer_Vibration_Amplitude  Frequency=LDW_Steer_Vibration_Freq*2*pi  SampleTime=0
  Logical Operator : Logic  Operator=OR  AllPortsSameDT=off  OutDataTypeStr=boolean
  Logical Operator1 : Logic  Inputs=7  AllPortsSameDT=off  OutDataTypeStr=boolean
  Logical Operator2 : Logic  AllPortsSameDT=off  OutDataTypeStr=boolean
  Logical Operator3 : Logic  AllPortsSameDT=off  OutDataTypeStr=boolean
  Logical Operator4 : Logic  Operator=OR  AllPortsSameDT=off  OutDataTypeStr=boolean
  Logical Operator5 : Logic  Inputs=3  AllPortsSameDT=off  OutDataTypeStr=boolean
  Memory2 : Memory
  Mux3 : Mux  Inputs=2
  Product : Product  Inputs=3
  Product1 : Product
  Product2 : Product
  Pulse Generator : DiscretePulseGenerator  PulseType=Time based  Period=1/LKA_On_Display_Freq  PulseWidth=50
  Rate Transition : RateTransition  OutPortSampleTime=1/LDW_Freq_Hz
  Rate Transition1 : RateTransition  OutPortSampleTime=1/1000
  Rate Transition2 : RateTransition  OutPortSampleTime=1/1000
  Rate Transition3 : RateTransition  OutPortSampleTime=1/1000
  Terminator : Terminator
  Terminator1 : Terminator
  tag scope: LDW_On=global, LDW_On_Left=global, LDW_On_Pulse=global, LDW_On_Right=global, LDW_Ready=global, LDW_Steering_Torque=global, LDW_White=global
  wires:
  [Vicrt_Status] -> Compare To Constant1/1
  Compare To Constant1/1 -> Logical Operator1/1
  Logical Operator1/1 -> Logical Operator3/1, Data Type Conversion/1  "trigger ldw"
  [Vehicle_Speed] -> Compare To LDW_Min_Speed/1
  Compare To LDW_Min_Speed/1 -> Logical Operator2/2, Logical Operator1/4
  Logical Operator/1 -> Logical Operator1/3
  LDW_Steer_Vibration/1 -> Product1/1
  Product1/1 -> Rate Transition3/1
  Data Type Conversion/1 -> Product2/1, [LDW_On], Product1/2
  Logical Operator2/1 -> Logical Operator5/1, Data Type Conversion1/1
  Data Type Conversion1/1 -> [LDW_White]
  Demux/1 -> Logical Operator/1
  Demux/2 -> Logical Operator/2
  Demux1/1 -> [LDW_On_Left]
  Demux1/2 -> [LDW_On_Right]
  Data Type Conversion3/1 -> Demux1/1
  Logical Operator3/1 -> Data Type Conversion3/1
  Rate Transition/1 -> Rate Transition1/1, Discrete Derivative/1
  Discrete Derivative/1 -> Abs/1
  Rate Transition2/1 -> Compare To LDW_LaneGap_dydt_Warning/1
  Compare To LDW_LaneGap_dydt_Warning/1 -> Demux2/1
  Logical Operator4/1 -> Logical Operator1/2
  Demux2/1 -> Logical Operator4/1
  Demux2/2 -> Logical Operator4/2
  Abs/1 -> Rate Transition2/1
  [Indicator_On] -> Compare To Constant4/1
  Compare To Constant4/1 -> Logical Operator1/6, Logical Operator5/2
  Logical Operator5/1 -> Data Type Conversion2/1
  Product/1 -> Logical Operator2/1, Logical Operator1/5  "aaaaaa"
  [ADAS_Error] -> Compare To Zero/1
  Compare To Zero/1 -> Product/1
  LDW_Activity_Flag/1 -> Product/2
  LDW_LaneGap_Warning1/1(Out1) -> Logical Operator3/2, Demux/1
  Rate Transition1/1 -> LDW_LaneGap_Warning1/1(In1)
  [AP_On] -> Memory2/1
  Memory2/1 -> Compare To Constant3/1
  Compare To Constant3/1 -> Logical Operator1/7, Logical Operator5/3
  Pulse Generator/1 -> Product2/2
  Product2/1 -> [LDW_On_Pulse]
  [LKA_On] -> Compare To Constant2/1
  Compare To Constant2/1 -> Terminator/1
  Rate Transition3/1 -> [LDW_Steering_Torque]
  Data Type Conversion2/1 -> [LDW_Ready]
  Mux3/1 -> Rate Transition/1
  [LaneGap_left_ws] -> Mux3/1
  [LaneGap_right_ws] -> Mux3/2
  [LSS_controls_Start_signal] -> Product/3
  Constant/1 -> [AP_On], [ADAS_Error], [Indicator_On]
  [LDW_Steering_Torque] -> Bus Creator/1
  [LDW_On] -> Bus Creator/2
  [LDW_On_Pulse] -> Bus Creator/3
  [LDW_On_Left] -> Bus Creator/4
  [LDW_On_Right] -> Bus Creator/5
  [LDW_White] -> Bus Creator/6
  [LDW_Ready] -> Bus Creator/7
  Bus Creator/1 -> Terminator1/1

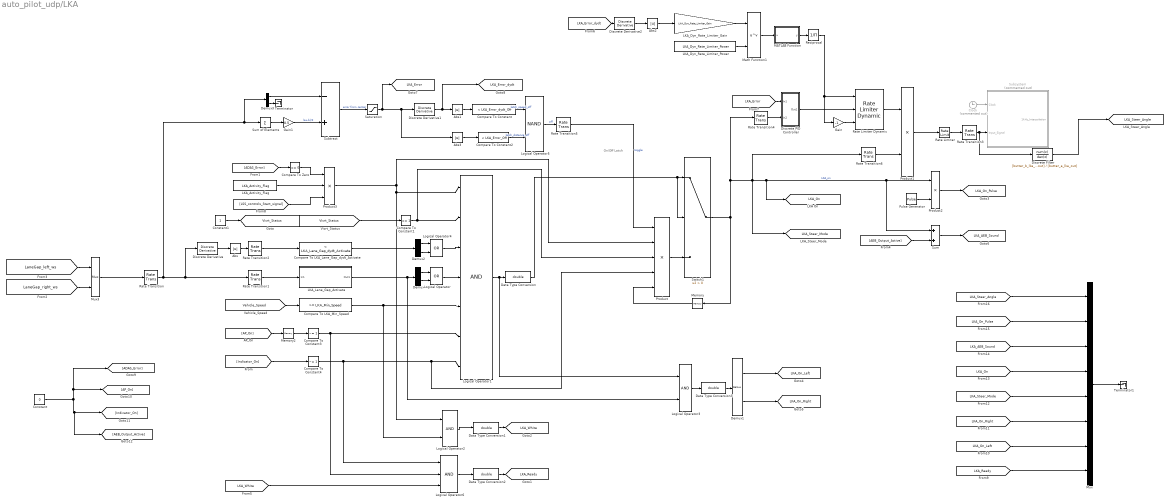
== system auto_pilot_udp/LKA ==
  note: On/Off Latch
  Abs{,1..3} (4 alike) : Abs  SaturateOnIntegerOverflow=off
  Clock : Clock  Commented=on
  Compare To Constant : simulink/Logic and Bit Operations/Compare To Constant  relop=<  const=LKA_Error_dydt_Off  OutDataTypeStr=boolean
  Compare To Constant1 : simulink/Logic and Bit Operations/Compare To Constant  relop===  const=1  OutDataTypeStr=boolean
  Compare To Constant2 : simulink/Logic and Bit Operations/Compare To Constant  relop=<  const=LKA_Error_Off  OutDataTypeStr=boolean
  Compare To Constant3 : simulink/Logic and Bit Operations/Compare To Constant  relop=~=  const=1  OutDataTypeStr=boolean
  Compare To Constant4 : simulink/Logic and Bit Operations/Compare To Constant  relop=~=  const=1  OutDataTypeStr=boolean
  Compare To LKA_Lane_Gap_dydt_Activate : simulink/Logic and Bit Operations/Compare To Constant  relop=<  const=LKA_Lane_Gap_dydt_Activate  OutDataTypeStr=boolean
  Compare To LKA_Min_Speed : simulink/Logic and Bit Operations/Compare To Constant  relop=>=  const=LKA_Min_Speed  OutDataTypeStr=boolean
  Compare To Zero : simulink/Logic and Bit Operations/Compare To Zero  relop===  OutDataTypeStr=boolean
  Constant : Constant  Value=0
  Constant1 : Constant
  Data Type Conversion{,1..3} (4 alike) : DataTypeConversion  OutDataTypeStr=double  SaturateOnIntegerOverflow=off  RndMeth=Floor
  Demux{,1..3} (4 alike) : Demux  Outputs=2
  Discrete Derivative : simulink/Discrete/Discrete Derivative  gainval=1.0  ICPrevScaledInput=0.0  OutMin=[]  OutMax=[]  OutDataType=fixdt(1, 16)  OutScaling=2^-10  DoSatur=off
  Discrete Derivative1 : simulink/Discrete/Discrete Derivative  gainval=1.0  ICPrevScaledInput=0.0  OutMin=[]  OutMax=[]  OutDataType=fixdt(1, 16)  OutScaling=2^-10  DoSatur=off
  Discrete Derivative2 : simulink/Discrete/Discrete Derivative  gainval=1.0  ICPrevScaledInput=0.0  OutMin=[]  OutMax=[]  OutDataType=fixdt(1, 16)  OutScaling=2^-10  DoSatur=off
  Discrete Filter : DiscreteFilter  Numerator=[butter_b_lka_out]  Denominator=[butter_a_lka_out]  SampleTime=1e-3
  Discrete PID Controller : Subsystem
  Gain : Gain  Gain=-1
  Gain1 : Gain  Gain=0.5
  LKA_Activity_Flag : Constant  Value=LKA_Activity_Flag
  LKA_Dyn_Rate_Limiter_Gain : Gain  Gain=LKA_Dyn_Rate_Limiter_Gain
  LKA_Dyn_Rate_Limiter_Power : Constant  Value=LKA_Dyn_Rate_Limiter_Power
  LKA_Lane_Gap_Activate : Subsystem
  Logical Operator : Logic  Operator=OR  AllPortsSameDT=off  OutDataTypeStr=boolean
  Logical Operator1 : Logic  Inputs=7  AllPortsSameDT=off  OutDataTypeStr=boolean
  Logical Operator2 : Logic  AllPortsSameDT=off  OutDataTypeStr=boolean
  Logical Operator3 : Logic  AllPortsSameDT=off  OutDataTypeStr=boolean
  Logical Operator4 : Logic  Operator=OR  AllPortsSameDT=off  OutDataTypeStr=boolean
  Logical Operator5 : Logic  Operator=NAND  AllPortsSameDT=off  OutDataTypeStr=boolean
  Logical Operator6 : Logic  Inputs=3  AllPortsSameDT=off  OutDataTypeStr=boolean
  MATLAB Function : MATLAB Function  TreatAsAtomicUnit=on
  Math Function1 : Math  Operator=pow  SignedPower=on
  Memory : Memory
  Memory2 : Memory
  Mux : Mux  Inputs=8
  Mux3 : Mux  Inputs=2
  Product : Product  Inputs=5
  Product1 : Product
  Product2 : Product
  Product3 : Product  Inputs=3
  Pulse Generator : DiscretePulseGenerator  PulseType=Time based  Period=1/LKA_On_Display_Freq  PulseWidth=50
  Rate Limiter : RateLimiter  RisingSlewLimit=LKA_Steer_Rate_Max_radps  FallingSlewLimit=-LKA_Steer_Rate_Max_radps  SampleTimeMode=inherited
  Rate Limiter Dynamic : simulink/Discontinuities/Rate Limiter Dynamic
  Rate Transition : RateTransition  OutPortSampleTime=1/LKA_Freq_Hz
  Rate Transition{1..3,5} (4 alike) : RateTransition  OutPortSampleTime=1/1000
  Rate Transition4 : RateTransition  OutPortSampleTime=1/LKA_Freq_Hz
  Rate Transition6 : RateTransition  OutPortSampleTime=1/LKA_Freq_Hz
  Reciprocal : Product  Inputs=/  RndMeth=Zero  SaturateOnIntegerOverflow=on
  Saturation : Saturate  UpperLimit=LKA_Error_Max  LowerLimit=-LKA_Error_Max
  Subsystem : Subsystem  Commented=on
  Subtract : Sum  Inputs=-+
  Sum : Sum
  Sum of Elements : Sum  Inputs=+
  Switch1 : Switch  Criteria=u2 > Threshold  SaturateOnIntegerOverflow=off  InputSameDT=off
  Terminator : Terminator
  Terminator1 : Terminator
  tag scope: LKA_AEB_Sound=global, LKA_Error=global, LKA_Error_dydt=global, LKA_On=global, LKA_On_Left=global, LKA_On_Pulse=global, LKA_On_Right=global, LKA_Ready=global, LKA_Steer_Angle=global, LKA_Steer_Mode=global, LKA_White=global, Vicrt_Status=global
  wires:
  [Vicrt_Status] -> Compare To Constant1/1
  Compare To Constant1/1 -> Product/3, Logical Operator1/2
  Logical Operator1/1 -> Logical Operator3/1, Data Type Conversion/1
  [Vehicle_Speed] -> Compare To LKA_Min_Speed/1
  Compare To LKA_Min_Speed/1 -> Logical Operator1/5, Logical Operator2/2
  Logical Operator/1 -> Logical Operator1/4
  Logical Operator2/1 -> Data Type Conversion1/1
  Data Type Conversion1/1 -> [LKA_White]
  Demux/1 -> Logical Operator/1
  Demux/2 -> Logical Operator/2
  LKA_Lane_Gap_Activate/1(Out1) -> Logical Operator3/2, Demux/1
  Data Type Conversion3/1 -> Demux1/1
  Logical Operator3/1 -> Data Type Conversion3/1
  Rate Transition/1 -> Demux3/1, Sum of Elements/1, Discrete Derivative/1, Rate Transition1/1
  Discrete Derivative/1 -> Abs/1
  Rate Transition1/1 -> LKA_Lane_Gap_Activate/1(In1)
  Rate Transition2/1 -> Compare To LKA_Lane_Gap_dydt_Activate/1
  Compare To LKA_Lane_Gap_dydt_Activate/1 -> Demux2/1
  Logical Operator4/1 -> Logical Operator1/3
  Demux2/1 -> Logical Operator4/1
  Demux2/2 -> Logical Operator4/2
  Abs/1 -> Rate Transition2/1
  Data Type Conversion/1 -> Switch1/1, Switch1/2
  Product/1 -> Switch1/3
  Memory/1 -> Product/5
  Logical Operator5/1 -> Rate Transition5/1  "off"
  Sum of Elements/1 -> Gain1/1
  Gain1/1 -> Subtract/2  "(a+b)/2"
  Demux3/2 -> Terminator/1
  Demux3/1 -> Subtract/1
  Subtract/1 -> Saturation/1  "error from center"
  Clock/1 -> Subsystem/1(Clock)
  Compare To Constant/1 -> Logical Operator5/1  "latch_speed_off"
  Compare To Constant2/1 -> Logical Operator5/2  "latch_distance_off"
  Rate Transition5/1 -> Product/1  "toggle"
  Gain/1 -> Rate Limiter Dynamic/3
  Rate Limiter Dynamic/1 -> Product1/1
  Rate Limiter/1 -> Rate Transition3/1
  LKA_Dyn_Rate_Limiter_Power/1 -> Math Function1/2
  Math Function1/1 -> MATLAB Function/1(u)
  LKA_Dyn_Rate_Limiter_Gain/1 -> Math Function1/1
  Reciprocal/1 -> Rate Limiter Dynamic/1, Gain/1
  Abs1/1 -> Compare To Constant/1
  Discrete Derivative2/1 -> Abs2/1
  Abs2/1 -> LKA_Dyn_Rate_Limiter_Gain/1
  Abs3/1 -> Compare To Constant2/1
  Saturation/1 -> Abs3/1, Discrete Derivative1/1, [LKA_Error]
  Product1/1 -> Rate Limiter/1
  Rate Transition6/1 -> Product1/2
  Discrete Derivative1/1 -> Abs1/1, [LKA_Error_dydt]
  Pulse Generator/1 -> Product2/2
  Rate Transition3/1 -> Discrete Filter/1, Subsystem/2(Input_Signal)
  Mux3/1 -> Rate Transition/1
  [AP_On] -> Memory2/1
  Compare To Constant3/1 -> Logical Operator1/6, Logical Operator6/2
  Memory2/1 -> Compare To Constant3/1
  [Indicator_On] -> Compare To Constant4/1
  Compare To Constant4/1 -> Product/4, Logical Operator1/7, Logical Operator6/1
  Data Type Conversion2/1 -> [LKA_Ready]
  Logical Operator6/1 -> Data Type Conversion2/1
  [ADAS_Error] -> Compare To Zero/1
  Compare To Zero/1 -> Product3/1
  Product3/1 -> Logical Operator2/1, Logical Operator1/1, Product/2
  Rate Transition4/1 -> Discrete PID Controller/2(In2)
  Discrete PID Controller/1(Out1) -> Rate Limiter Dynamic/2
  Switch1/1 -> Rate Transition6/1, [LKA_Steer_Mode], [LKA_On], Sum/1, Product2/1, Rate Transition4/1, Memory/1  "LKA_on"
  [AEB_Output_Active] -> Sum/2
  Product2/1 -> [LKA_On_Pulse]
  Demux1/1 -> [LKA_On_Left]
  Demux1/2 -> [LKA_On_Right]
  Sum/1 -> [LKA_AEB_Sound]
  [LaneGap_right_ws] -> Mux3/2
  [LaneGap_left_ws] -> Mux3/1
  [LKA_White] -> Logical Operator6/3
  [LKA_Error_dydt] -> Discrete Derivative2/1
  [LKA_Error] -> Discrete PID Controller/1(In1)
  Constant1/1 -> [Vicrt_Status]
  Discrete Filter/1 -> [LKA_Steer_Angle]
  LKA_Activity_Flag/1 -> Product3/2
  [LSS_controls_Start_signal] -> Product3/3
  Constant/1 -> [AEB_Output_Active], [Indicator_On], [AP_On], [ADAS_Error]
  [LKA_Steer_Angle] -> Mux/1
  [LKA_On_Pulse] -> Mux/2
  [LKA_AEB_Sound] -> Mux/3
  [LKA_On] -> Mux/4
  [LKA_Steer_Mode] -> Mux/5
  [LKA_On_Right] -> Mux/6
  [LKA_On_Left] -> Mux/7
  [LKA_Ready] -> Mux/8
  Mux/1 -> Terminator1/1
  MATLAB Function/1(y) -> Reciprocal/1

== system auto_pilot_udp/OUTPUT ==
  VI-CarRealTime_Outputs : Subsystem
  VI-CarRealTime_Outputs2 : Subsystem  Commented=on
  WorldSim_Sensor_Outputs : Subsystem
  rough data reporting : Subsystem

== system auto_pilot_udp/STOP manager ==
  Clock2 : Clock
  Compare To Constant : simulink/Logic and Bit Operations/Compare To Constant  relop=>  const=stop_time  OutDataTypeStr=boolean
  Compare To Constant1 : simulink/Logic and Bit Operations/Compare To Constant  relop=<=  const=stop_speed  OutDataTypeStr=boolean
  Compare To Constant2 : simulink/Logic and Bit Operations/Compare To Constant  relop=>=  const=stop_number_collisions  OutDataTypeStr=boolean
  Constant : Constant  Value=0
  OR : Logic  Operator=OR  Inputs=4  AllPortsSameDT=off  OutDataTypeStr=boolean
  Stop Simulation : Stop
  wires:
  [collision_additive] -> Compare To Constant2/1
  Compare To Constant2/1 -> OR/3
  Compare To Constant/1 -> OR/1
  [Vehicle_Speed] -> Compare To Constant1/1
  Clock2/1 -> Compare To Constant/1
  Compare To Constant1/1 -> OR/2
  OR/1 -> Stop Simulation/1
  [LKA_Stop_signal] -> OR/4
  Constant/1 -> [LKA_Stop_signal]

== system auto_pilot_udp/SteeringButtonsMap ==
  VI_DriveSim.Inputs.Control.VICRT_RESTART_REQ : simwbSfunlib/toRTDBc  Commented=on  stringBlock=off  varName=VI_DriveSim.Inputs.Control.VICRT_RESTART_REQ  sigDim=[1 1]  sigType=double  sampleTime=[-1 0]  maxBuffSize=1024  busName=nobus  defaultValue=0  defaultString=simwbout  hasMapping=0  ptrName=VI_DriveSim_Inputs_Control_VICRT_RESTART_REQ  enumOrAlias=nothing
      settings: SourceProductName=SimWB MLToolkit
  VI_DriveSim.Inputs.Control.VICRT_RESTORE_REQ : simwbSfunlib/toRTDBc  stringBlock=off  varName=VI_DriveSim.Inputs.Control.VICRT_RESTORE_REQ  sigDim=[1 1]  sigType=double  sampleTime=[-1 0]  maxBuffSize=1024  busName=nobus  defaultValue=0  defaultString=simwbout  hasMapping=0  ptrName=VI_DriveSim_Inputs_Control_VICRT_RESTORE_REQ  enumOrAlias=nothing
      settings: SourceProductName=SimWB MLToolkit
  VI_DriveSim.Inputs.ECAT.BECKH.DIG3 : simwbSfunlib/fromRTDBc  stringBlock=off  varName=VI_DriveSim.Inputs.ECAT.BECKH.DIG3  sigDim=[1 1]  sigType=double  sampleTime=[-1 0]  maxBuffSize=1024  busName=nobus  defaultValue=0  defaultString=simwbin  hasMapping=0  ptrName=VI_DriveSim_Inputs_ECAT_BECKH_DIG3  enumOrAlias=nothing
      settings: SourceProductName=SimWB MLToolkit
  VI_DriveSim.Inputs.ECAT.BECKH.DIG4 : simwbSfunlib/fromRTDBc  stringBlock=off  varName=VI_DriveSim.Inputs.ECAT.BECKH.DIG4  sigDim=[1 1]  sigType=double  sampleTime=[-1 0]  maxBuffSize=1024  busName=nobus  defaultValue=0  defaultString=simwbin  hasMapping=0  ptrName=VI_DriveSim_Inputs_ECAT_BECKH_DIG4  enumOrAlias=nothing
      settings: SourceProductName=SimWB MLToolkit
  tag scope: ADAS_Request=global
  wires:
  VI_DriveSim.Inputs.ECAT.BECKH.DIG3/1 -> VI_DriveSim.Inputs.Control.VICRT_RESTORE_REQ/1
  VI_DriveSim.Inputs.ECAT.BECKH.DIG4/1 -> [ADAS_Request], VI_DriveSim.Inputs.Control.VICRT_RESTART_REQ/1
